simulink model "DEKFSensorless"  (R2019b)
settings: Solver=VariableStepAuto  StartTime=0.0  StopTime=1  RelTol=1e-3
undefined symbols (not defined in the file): DiscIntNeverNeededParam, Fh, Id0, InitParam, inv_L, Iq0, J, L, Psi_dm, Qp, Qx, R, Rs, Tilde_theta, Tsim, Ud0, Umd, Umq, Uq0, we
settings Model: SimulationMode=accelerator  Creator=Downstream  LastModifiedBy=Downstream

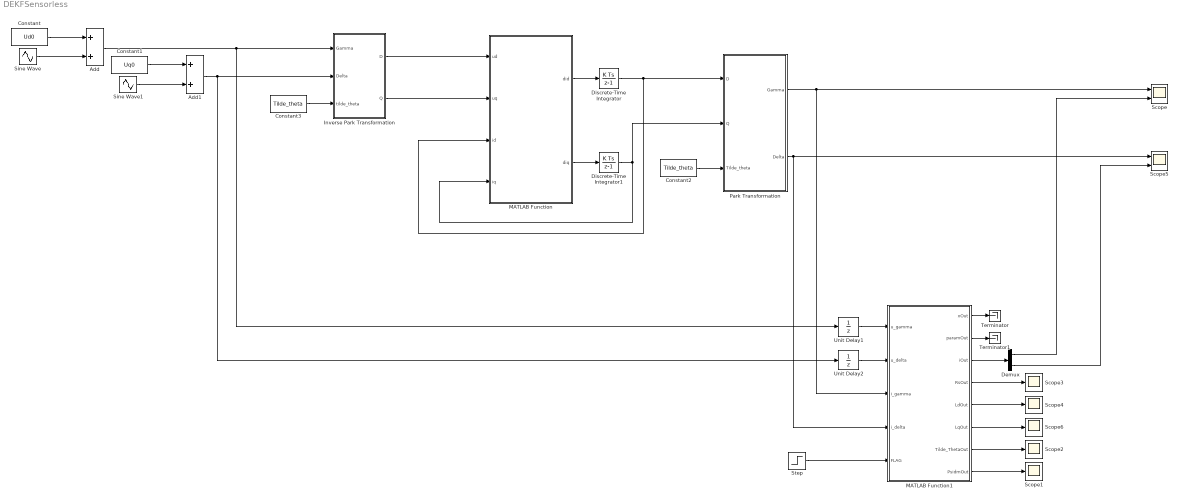
== system DEKFSensorless ==
  Add : Sum
  Add1 : Sum
  Constant : Constant  Value=Ud0  SampleTime=Tsim
  Constant1 : Constant  Value=Uq0  SampleTime=Tsim
  Constant2 : Constant  Value=Tilde_theta  SampleTime=-1
  Constant3 : Constant  Value=Tilde_theta  SampleTime=-1
  Demux : Demux  Outputs=2
  Discrete-Time Integrator : DiscreteIntegrator  InitialCondition=Id0  SampleTime=Tsim  ICPrevOutput=DiscIntNeverNeededParam  ICPrevScaledInput=DiscIntNeverNeededParam
  Discrete-Time Integrator1 : DiscreteIntegrator  InitialCondition=Iq0  SampleTime=Tsim  ICPrevOutput=DiscIntNeverNeededParam  ICPrevScaledInput=DiscIntNeverNeededParam
  Inverse Park Transformation : Subsystem
  MATLAB Function : MATLAB Function  TreatAsAtomicUnit=on
  MATLAB Function1 : MATLAB Function  TreatAsAtomicUnit=on  SystemSampleTime=Tsim
  Park Transformation : Subsystem
  Scope : Scope  NumInputPorts=2
  Scope{1..4,6} (5 alike) : Scope
  Scope5 : Scope  NumInputPorts=2
  Sine Wave : Sin  Amplitude=Umd  Frequency=Fh*2*pi  SampleTime=Tsim
  Sine Wave1 : Sin  Amplitude=Umq  Frequency=Fh*2*pi  Phase=pi/2  SampleTime=Tsim
  Step : Step  Time=0.2  SampleTime=Tsim
  Terminator : Terminator
  Terminator1 : Terminator
  Unit Delay1 : UnitDelay  SampleTime=-1  HasFrameUpgradeWarning=on
  Unit Delay2 : UnitDelay  SampleTime=-1  HasFrameUpgradeWarning=on
  wires:
  MATLAB Function/1(did) -> Discrete-Time Integrator/1
  MATLAB Function/2(diq) -> Discrete-Time Integrator1/1
  Discrete-Time Integrator/1 -> Park Transformation/1(D), MATLAB Function/3(id)
  Discrete-Time Integrator1/1 -> MATLAB Function/4(iq), Park Transformation/2(Q)
  Inverse Park Transformation/1(D) -> MATLAB Function/1(ud)
  Inverse Park Transformation/2(Q) -> MATLAB Function/2(uq)
  Constant2/1 -> Park Transformation/3(Tilde_theta)
  Constant3/1 -> Inverse Park Transformation/3(tilde_theta)
  Constant/1 -> Add/1
  Constant1/1 -> Add1/1
  Sine Wave/1 -> Add/2
  Sine Wave1/1 -> Add1/2
  Demux/1 -> Scope/2
  Demux/2 -> Scope5/2
  MATLAB Function1/3(iOut) -> Demux/1
  MATLAB Function1/4(RsOut) -> Scope3/1
  MATLAB Function1/5(LdOut) -> Scope4/1
  MATLAB Function1/6(LqOut) -> Scope6/1
  MATLAB Function1/8(PsidmOut) -> Scope1/1
  Step/1 -> MATLAB Function1/5(FLAG)
  Add1/1 -> Unit Delay2/1, Inverse Park Transformation/2(Delta)
  Add/1 -> Unit Delay1/1, Inverse Park Transformation/1(Gamma)
  Park Transformation/1(Gamma) -> MATLAB Function1/3(i_gamma), Scope/1
  Park Transformation/2(Delta) -> MATLAB Function1/4(i_delta), Scope5/1
  Unit Delay1/1 -> MATLAB Function1/1(u_gamma)
  Unit Delay2/1 -> MATLAB Function1/2(u_delta)
  MATLAB Function1/7(Tilde_ThetaOut) -> Scope2/1
  MATLAB Function1/1(xOut) -> Terminator/1
  MATLAB Function1/2(paramOut) -> Terminator1/1

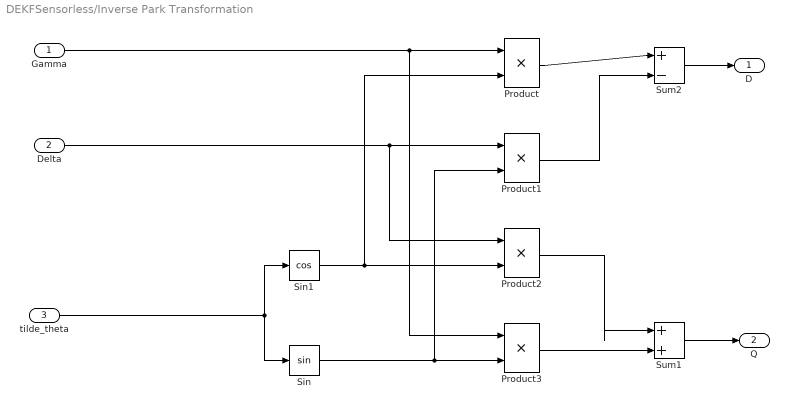
== system DEKFSensorless/Inverse Park Transformation ==
  Gamma : Inport
  Delta : Inport  Port=2
  tilde_theta : Inport  Port=3
  Product{,1..3} (4 alike) : Product  OutDataTypeStr=Inherit: Same as first input
  Sin : Trigonometry  OutputSignalType=real
  Sin1 : Trigonometry  Operator=cos  OutputSignalType=real
  Sum1 : Sum  Inputs=|++  OutDataTypeStr=Inherit: Same as first input
  Sum2 : Sum  Inputs=|+-  OutDataTypeStr=Inherit: Same as first input
  D : Outport
  Q : Outport  Port=2
  wires:
  Sin1/1 -> Product2/2, Product/2
  Sin/1 -> Product3/2, Product1/2
  Product3/1 -> Sum1/2
  Sum1/1 -> Q/1
  Gamma/1 -> Product3/1, Product/1
  Product2/1 -> Sum1/1
  Sum2/1 -> D/1
  Product/1 -> Sum2/1
  Product1/1 -> Sum2/2
  Delta/1 -> Product2/1, Product1/1
  tilde_theta/1 -> Sin/1, Sin1/1

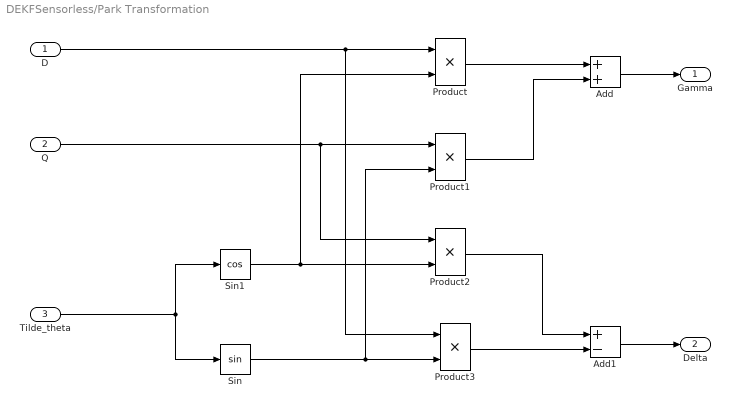
== system DEKFSensorless/Park Transformation ==
  D : Inport
  Q : Inport  Port=2
  Tilde_theta : Inport  Port=3
  Add : Sum
  Add1 : Sum  Inputs=+-
  Product{,1..3} (4 alike) : Product
  Sin : Trigonometry  OutputSignalType=real
  Sin1 : Trigonometry  Operator=cos  OutputSignalType=real
  Gamma : Outport
  Delta : Outport  Port=2
  wires:
  Product/1 -> Add/1
  Sin/1 -> Product3/2, Product1/2
  Product1/1 -> Add/2
  Add1/1 -> Delta/1
  Sin1/1 -> Product2/2, Product/2
  Product2/1 -> Add1/1
  D/1 -> Product3/1, Product/1
  Q/1 -> Product2/1, Product1/1
  Product3/1 -> Add1/2
  Add/1 -> Gamma/1
  Tilde_theta/1 -> Sin/1, Sin1/1

== matlab function DEKFSensorless/MATLAB Function1 ==
  data: u_gamma input; xOut output; u_delta input; i_gamma input; i_delta input; Qp parameter; we parameter; J parameter; Qx parameter; R parameter; paramOut output; iOut output; RsOut output; LdOut output; LqOut output; Tilde_ThetaOut output; PsidmOut output; FLAG input; Tsim parameter; InitParam parameter
function [xOut,paramOut,iOut,RsOut,LdOut,LqOut,Tilde_ThetaOut,PsidmOut] = DEKF(u_gamma,u_delta,i_gamma,i_delta,Qp, we, J, Qx, R, FLAG,Tsim,InitParam)
u = [u_gamma;u_delta;];
i = [i_gamma;i_delta;];
% Tsim = 1e-4;
% InitPercent = 0.5;
persistent hat_x hat_param P_hat_x P_hat_param;
if isempty(hat_x)
    hat_x = [0;0;];
%     hat_param = [0.8;1/1.6e-3;0;1/3.2e-3;0.047;] * InitPercent;
    hat_param = InitParam;
    P_hat_x = zeros(2);
    P_hat_param = zeros(5);
end



persistent difx_difparam K_xk_1 difH_difparam;
if isempty(difx_difparam)
    difx_difparam = zeros(2,5);
    K_xk_1 = zeros(2,2);
    difH_difparam = zeros(2,5);
end
%Step1: Parameter Prior Estimation
param_PE = hat_param;
P_param_PE = P_hat_param + Qp;
%Step2: State Prior Estimation
Rs = param_PE(1);
Ngg = param_PE(2); Ngd = param_PE(3); Ndd = param_PE(4);
Psidm = param_PE(5);
N = [Ngg Ngd;Ngd Ndd;];
A = (Rs * N + we * J);
tilde_theta = 1/2 * atan(-2 * Ngd / (Ndd - Ngg));
dot_x = u - A * hat_x - we * J * Psidm * [cos(tilde_theta);sin(tilde_theta);];
x_PE = hat_x + dot_x * Tsim;

A_dis = eye(2) - A * Tsim;
P_x_PE = A_dis * P_hat_x * A_dis' + Qx;
%step3: State Kalman Gain
K_xk = P_x_PE * N' * (N * P_x_PE * N' + R)^-1;
P_hat_x = (eye(2) - K_xk * N) * P_x_PE;
%Step4: Param Kalman Gain
difhat_x_difparam = difx_difparam - K_xk_1 * difH_difparam;

C1 = we * Psidm * cos(tilde_theta) * (1 * 1/(1 + (-2 * Ngd / (Ndd - Ngg))^2)) * (Ngd/((Ndd - Ngg)^2));
C2 = we * Psidm * sin(tilde_theta) * (1 * 1/(1 + (-2 * Ngd / (Ndd - Ngg))^2)) * (Ngd/((Ndd - Ngg)^2));

C3 = we * Psidm * cos(tilde_theta) * (1 * 1/(1 + (-2 * Ngd / (Ndd - Ngg))^2)) * (1/(Ndd - Ngg));
C4 = we * Psidm * sin(tilde_theta) * (1 * 1/(1 + (-2 * Ngd / (Ndd - Ngg))^2)) * (1/(Ndd - Ngg));

C5 = we * Psidm * cos(tilde_theta) * (1 * 1/(1 + (-2 * Ngd / (Ndd - Ngg))^2)) * (-Ngd/((Ndd - Ngg)^2));
C6 = we * Psidm * sin(tilde_theta) * (1 * 1/(1 + (-2 * Ngd / (Ndd - Ngg))^2)) * (-Ngd/((Ndd - Ngg)^2));

difG_difparam     = -Tsim * [Ngg * hat_x(1) + Ngd * hat_x(2), Rs * hat_x(1) + C1, Rs * hat_x(2) + C3, 0 + C5            , -we * sin(tilde_theta);...
                             Ngd * hat_x(1) + Ndd * hat_x(2), 0             + C2, Rs * hat_x(1) + C4, Rs * hat_x(2) + C6,  we * cos(tilde_theta);];
difG_difparam = difG_difparam + A_dis * difhat_x_difparam;
H_pk = [0, hat_x(1), hat_x(2), 0       , 0;...
        0, 0       , hat_x(1), hat_x(2), 0;];
H_pk = H_pk + N * difG_difparam;

K_pk = P_param_PE * H_pk' * (H_pk * P_param_PE * H_pk' + R)^-1;
P_hat_param = (eye(5) - K_pk * H_pk) * P_param_PE;
%step5: State & Param Prediction
hat_x = x_PE + K_xk * (i - N * x_PE);
hat_param = param_PE + K_pk * (i - N * x_PE);
if(hat_param(1) > 1.6)
    hat_param(1) = 1.6;
elseif(hat_param(1) < 0.4)
    hat_param(1) = 0.4;
end

if(hat_param(2) > 1/1.6e-3*10)
    hat_param(2) = 1/1.6e-3*10;
elseif(hat_param(2) < 1/1.6e-3/10)
    hat_param(2) = 1/1.6e-3/10;
end


if(hat_param(3) > 1/1.6e-3)
    hat_param(3) = 1/1.6e-3;
elseif(hat_param(3) < -1/1.6e-3)
    hat_param(3) = -1/1.6e-3;
end


if(hat_param(4) > 1/3.2e-3*10)
    hat_param(4) = 1/3.2e-3*10;
elseif(hat_param(4) < 1/3.2e-3/10)
    hat_param(4) = 1/3.2e-3/10;
end

if(hat_param(5) > 0.047 * 2)
    hat_param(5) = 0.047*2;
elseif(hat_param(5) < 0.047/2)
    hat_param(5) = 0.047/2;
end
% 
% if(hat_param(5) > 0.47)
%     hat_param(5) = 0.47;
% elseif(hat_param(5) < 0.47)
%     hat_param(5) = 0.47;
% end


%Step6: Update the parameter kalman gain
difx_difparam = difG_difparam;
K_xk_1 = K_xk;
difH_difparam = H_pk;

%Final: Output the results
if(FLAG == 0)
%     hat_param = [0.8;1/1.6e-3;0;1/3.2e-3;0.047;] * InitPercent;
    hat_param = InitParam;
    NOut = [hat_param(2) hat_param(3);hat_param(3) hat_param(4);];
    LOut = NOut^-1;
    hat_x = LOut * i;
    difx_difparam = zeros(2,5);
    K_xk_1 = zeros(2,2);
    difH_difparam = zeros(2,5);
end

xOut = hat_x;
NOut = [hat_param(2) hat_param(3);hat_param(3) hat_param(4);];
iOut = NOut * xOut;
paramOut = hat_param;
LOut = NOut^-1;
RsOut = hat_param(1);

Tilde_ThetaOut = 1/2 * atan(-2 * LOut(1,2)/(LOut(1,1)-LOut(2,2)));

P = [cos(Tilde_ThetaOut) sin(Tilde_ThetaOut);-sin(Tilde_ThetaOut) cos(Tilde_ThetaOut);];
LdqOut = P^-1 * LOut * P;
LdOut = LdqOut(1,1);
LqOut = LdqOut(2,2);
PsidmOut = hat_param(5);

== matlab function DEKFSensorless/MATLAB Function ==
  data: ud input; did output; uq input; id input; iq input; Rs parameter; L parameter; Psi_dm parameter; J parameter; we parameter; inv_L parameter; diq output
function [did,diq] = IPMSMLinearModel(ud,uq,id,iq,Rs, L, Psi_dm, J, we, inv_L)
u = [ud;uq;];
i = [id;iq;];
di = inv_L * (u - (Rs * eye(2) + we * J * L) * i - we * J * [Psi_dm;0;]);
did = di(1);
diq = di(2);
